simulink model "anti lock braking_system"  (R2024b)
settings: Solver=VariableStepAuto  StartTime=0.0  StopTime=30  RelTol=1e-3
model workspace (MAT data in the model file):
  R = 1.25
undefined symbols (not defined in the file): g, I, m, v0
settings Model: Creator=vaibh  LastModifiedBy=vaibh

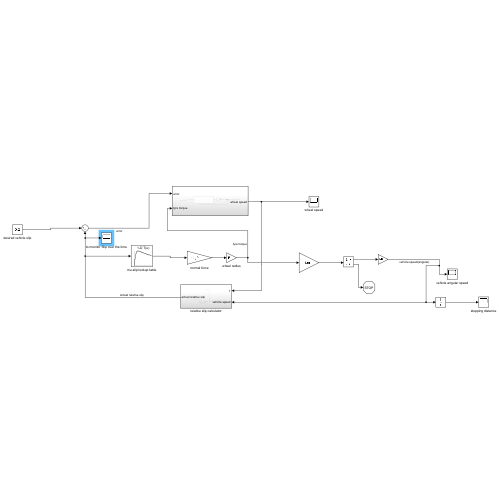
[thumbnail: Simulink's stored preview of the top-level diagram]
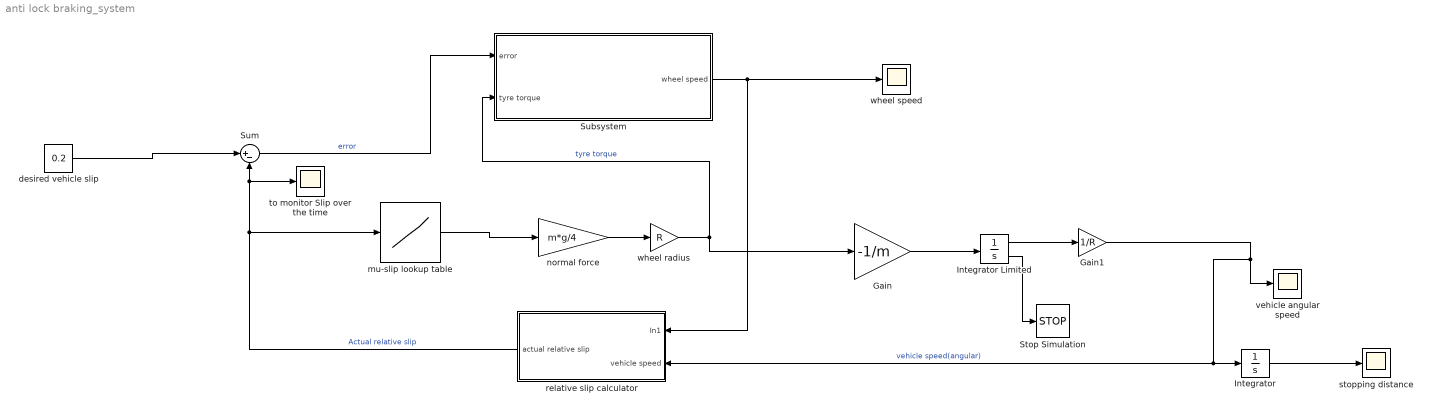
== system anti lock braking_system ==
  Gain : Gain  Gain=-1/m
  Gain1 : Gain  Gain=1/R
  Integrator : Integrator
  Integrator Limited : Integrator  InitialCondition=v0  LimitOutput=on  UpperSaturationLimit=1000  LowerSaturationLimit=0  ShowSaturationPort=on
  Stop Simulation : Stop
  Subsystem : Subsystem
  Sum : Sum  Inputs=|+-
  desired vehicle slip : Constant  Value=0.2
  mu-slip lookup table : Lookup_n-D  NumberOfTableDimensions=1  BreakpointsForDimension1=[0;0.050000000000000003;0.10000000000000001;0.14999999999999999;0.20000000000000001;0.25;0.29999999999999999;0.34999999999999998;0.40000000000000002;0.45000000000000001;0.5;0.55000000000000004;0.59999999999999998;0.65000000000000002;0.69999999999999996;0.75;0.80000000000000004;0.84999999999999998;0.90000000000000002;0.94999999999999996;1]  Table=[0;0.40000000000000002;0.80000000000000004;0.96999999999999997;1;0.97999999999999998;0.95999999999999996;0.93999999999999995;0.92000000000000004;0.90000000000000002;0.88;0.85499999999999998;0.82999999999999996;0.81000000000000005;0.79000000000000004;0.77000000000000002;0.75;0.72999999999999998;0.71999999999999997;0.70999999999999996;0.69999999999999996]  InternalRulePriority=Speed  RndMeth=Simplest
  normal force : Gain  Gain=m*g/4
  relative slip calculator : Subsystem
  stopping distance : Scope
  to monitor Slip over the time : Scope
  vehicle angular speed : Scope
  wheel radius : Gain  Gain=R
  wheel speed : Scope
  wires:
  desired vehicle slip/1 -> Sum/1
  mu-slip lookup table/1 -> normal force/1
  normal force/1 -> wheel radius/1
  Sum/1 -> Subsystem/1(error)  "error"
  wheel radius/1 -> Gain/1, Subsystem/2(tyre torque)  "tyre torque"
  Subsystem/1(wheel speed) -> wheel speed/1, relative slip calculator/1(In1)
  Gain/1 -> Integrator Limited/1
  Integrator Limited/1 -> Gain1/1
  Gain1/1 -> Integrator/1, relative slip calculator/2(vehicle speed), vehicle angular speed/1  "vehicle speed(angular)"
  Integrator Limited/2 -> Stop Simulation/1
  Integrator/1 -> stopping distance/1
  relative slip calculator/1(actual relative slip) -> mu-slip lookup table/1, to monitor Slip over the time/1, Sum/2  "Actual relative slip"

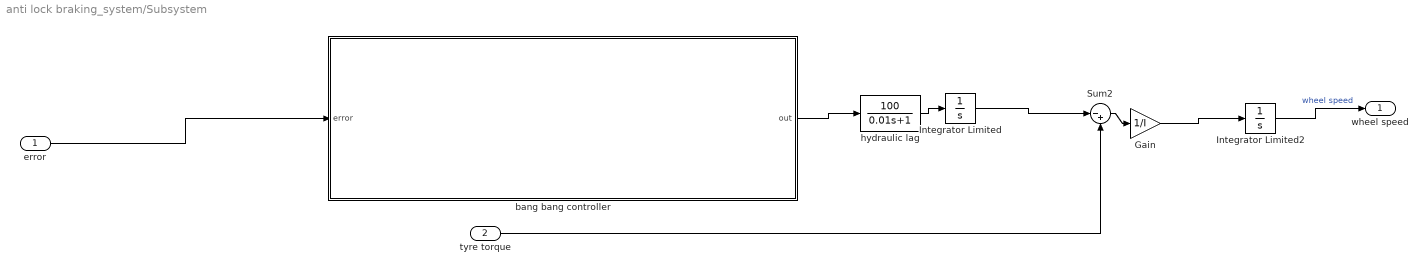
== system anti lock braking_system/Subsystem ==
  error : Inport
  tyre torque : Inport  Port=2
  " hydraulic lag" : TransferFcn  Numerator=[100]  Denominator=[0.01 1]
  Gain : Gain  Gain=1/I
  Integrator Limited : Integrator  LimitOutput=on  UpperSaturationLimit=1000  LowerSaturationLimit=0
  Integrator Limited2 : Integrator  InitialCondition=v0/R  LimitOutput=on  UpperSaturationLimit=1000  LowerSaturationLimit=0
  Sum2 : Sum  Inputs=|-+
  "bang bang controller " : Subsystem
  wheel speed : Outport
  wires:
  Gain/1 -> Integrator Limited2/1
  "bang bang controller "/1(out) -> " hydraulic lag"/1
  tyre torque/1 -> Sum2/2
  error/1 -> "bang bang controller "/1(error)
  " hydraulic lag"/1 -> Integrator Limited/1
  Sum2/1 -> Gain/1
  Integrator Limited2/1 -> wheel speed/1  "wheel speed"
  Integrator Limited/1 -> Sum2/1

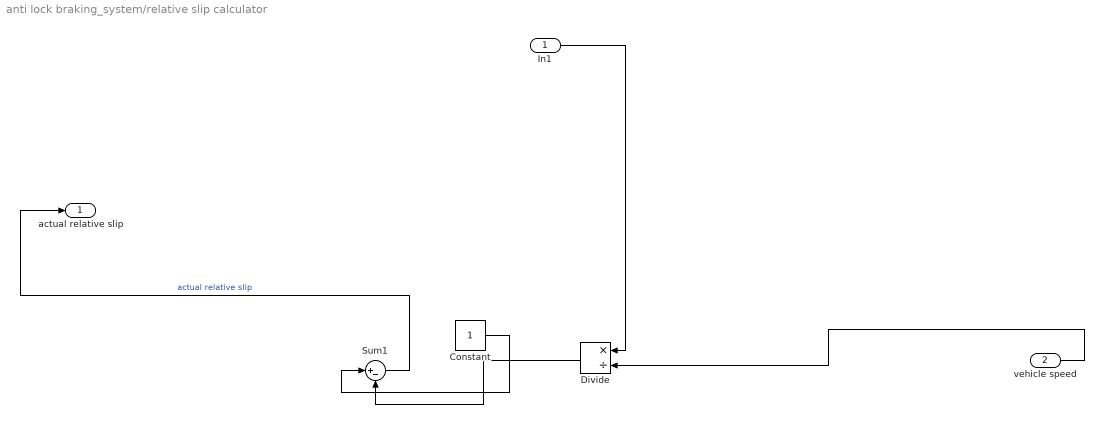
== system anti lock braking_system/relative slip calculator ==
  In1 : Inport
  vehicle speed : Inport  Port=2
  Constant : Constant
  Divide : Product  Inputs=*/
  Sum1 : Sum  Inputs=|+-
  actual relative slip : Outport
  wires:
  Divide/1 -> Sum1/2
  Constant/1 -> Sum1/1
  In1/1 -> Divide/1
  vehicle speed/1 -> Divide/2
  Sum1/1 -> actual relative slip/1  "actual relative slip"

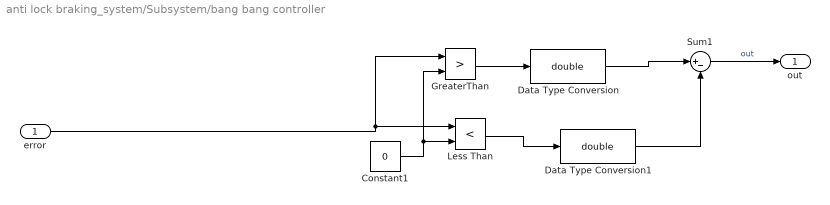
== system anti lock braking_system/Subsystem/bang bang controller  ==
  error : Inport
  Constant1 : Constant  Value=0
  Data Type Conversion : DataTypeConversion  OutDataTypeStr=double  SaturateOnIntegerOverflow=off
  Data Type Conversion1 : DataTypeConversion  OutDataTypeStr=double  SaturateOnIntegerOverflow=off
  GreaterThan : RelationalOperator  Operator=>  OutDataTypeStr=boolean  RndMeth=Simplest  InputSameDT=off
  Less Than : RelationalOperator  Operator=<  OutDataTypeStr=boolean  RndMeth=Simplest  InputSameDT=off
  Sum1 : Sum  Inputs=|+-
  out : Outport
  wires:
  Constant1/1 -> Less Than/2, GreaterThan/2
  Data Type Conversion/1 -> Sum1/1
  GreaterThan/1 -> Data Type Conversion/1
  error/1 -> GreaterThan/1, Less Than/1
  Data Type Conversion1/1 -> Sum1/2
  Less Than/1 -> Data Type Conversion1/1
  Sum1/1 -> out/1  "out"
